simulink model "controlGPI_pos_2dof_conMI"  (R2023b)
settings: Solver=ode45  StartTime=0.0  StopTime=tsim  FixedStep=5e-4  MaxStep=tstep
undefined symbols (not defined in the file): contr_robot_params, ddq, dq, MI_Contr1, MI_Contr2, MI_motor1, MI_motor2, ndof, NN_Bspline_params, NN_RBF_params, nn_select, ns, Pc, q, q0, q_cero, q_eq, robot_params, t_qeq_init, t_tr_init, t_trtr, tau_L, tau_L_mags, tr_muestra, Wc, Zc
libraries: mcbcontrolslib x4, spsRMSLib x4, simulink x2
(part 1 of 2)
settings Model: Creator=HP  LastModifiedBy=HP

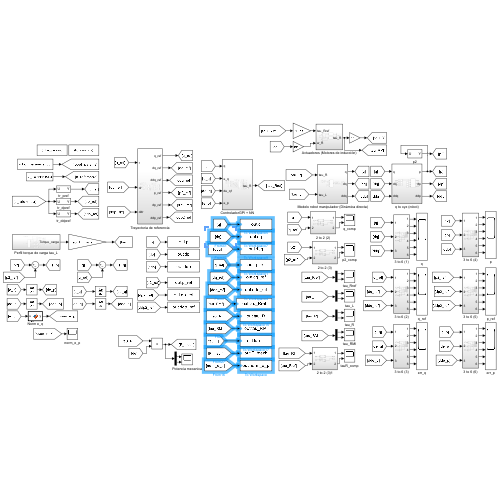
[thumbnail: Simulink's stored preview of the top-level diagram]
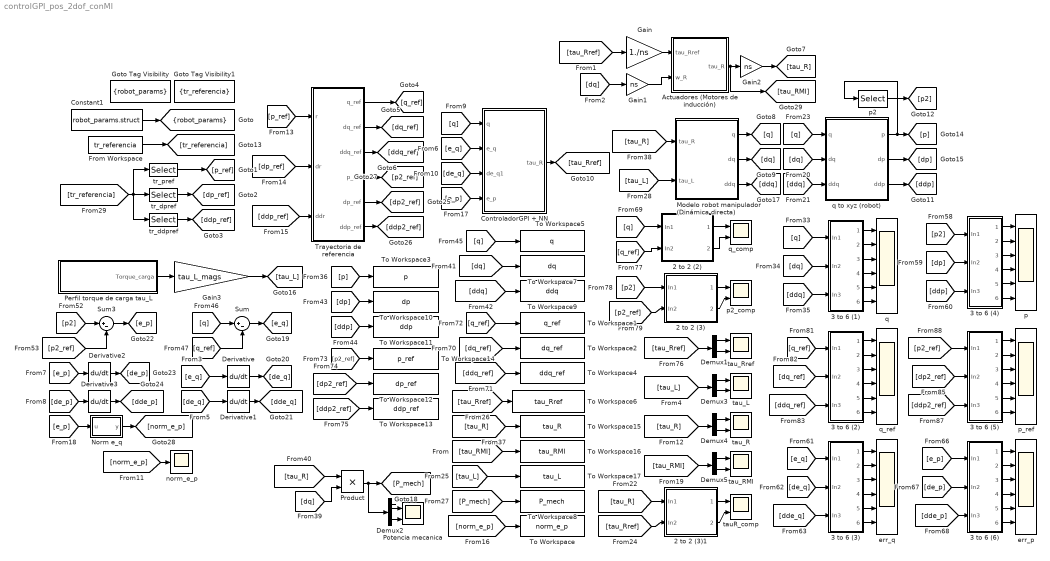
== system controlGPI_pos_2dof_conMI ==
  2 to 2 (2) : Subsystem
  2 to 2 (3) : Subsystem
  2 to 2 (3)1 : Subsystem
  3 to 6 (1) : Subsystem
  3 to 6 (2) : Subsystem
  3 to 6 (3) : Subsystem
  3 to 6 (4) : Subsystem
  3 to 6 (5) : Subsystem
  3 to 6 (6) : Subsystem
  Actuadores (Motores de inducción) : Subsystem
  Constant1 : Constant  Value=robot_params.struct  OutDataTypeStr=Bus: robot_params_bus
  ControladorGPI + NN : Subsystem
  Demux{1..5} (5 alike) : Demux  Outputs=2
  Derivative{,1..3} (4 alike) : Derivative
  From Workspace : FromWorkspace  VariableName=tr_referencia
  Gain : Gain  Gain=1./ns
  Gain1 : Gain  Gain=ns
  Gain2 : Gain  Gain=ns
  Gain3 : Gain  Gain=tau_L_mags
  Goto Tag Visibility : GotoTagVisibility  GotoTag=robot_params
  Goto Tag Visibility1 : GotoTagVisibility  GotoTag=tr_referencia
  Modelo robot manipulador (Dinámica directa) : Subsystem
  Norm e_q : MATLAB Function  TreatAsAtomicUnit=on
  Perfil torque de carga tau_L : Subsystem
  Potencia mecanica : Scope  NumInputPorts=2
  Product : Product
  Sum : Sum  Inputs=|+-
  Sum3 : Sum  Inputs=|+-
  To Workspace : ToWorkspace  VariableName=norm_e_p  SaveFormat=Timeseries  SampleTime=-1
  To Workspace1 : ToWorkspace  VariableName=q_ref  SaveFormat=Timeseries  SampleTime=-1
  To Workspace10 : ToWorkspace  VariableName=dp  SaveFormat=Timeseries  SampleTime=-1
  To Workspace11 : ToWorkspace  VariableName=ddp  SaveFormat=Timeseries  SampleTime=-1
  To Workspace12 : ToWorkspace  VariableName=dp_ref  SaveFormat=Timeseries  SampleTime=-1
  To Workspace13 : ToWorkspace  VariableName=ddp_ref  SaveFormat=Timeseries  SampleTime=-1
  To Workspace14 : ToWorkspace  VariableName=p_ref  SaveFormat=Timeseries  SampleTime=-1
  To Workspace15 : ToWorkspace  VariableName=tau_R  SaveFormat=Timeseries  SampleTime=-1
  To Workspace16 : ToWorkspace  VariableName=tau_RMI  SaveFormat=Timeseries  SampleTime=-1
  To Workspace17 : ToWorkspace  VariableName=tau_L  SaveFormat=Timeseries  SampleTime=-1
  To Workspace2 : ToWorkspace  VariableName=dq_ref  SaveFormat=Timeseries  SampleTime=-1
  To Workspace3 : ToWorkspace  VariableName=p  SaveFormat=Timeseries  SampleTime=-1
  To Workspace4 : ToWorkspace  VariableName=ddq_ref  SaveFormat=Timeseries  SampleTime=-1
  To Workspace5 : ToWorkspace  VariableName=q  SaveFormat=Timeseries  SampleTime=-1
  To Workspace6 : ToWorkspace  VariableName=tau_Rref  SaveFormat=Timeseries  SampleTime=-1
  To Workspace7 : ToWorkspace  VariableName=dq  SaveFormat=Timeseries  SampleTime=-1
  To Workspace8 : ToWorkspace  VariableName=P_mech  SaveFormat=Timeseries  SampleTime=-1
  To Workspace9 : ToWorkspace  VariableName=ddq  SaveFormat=Timeseries  SampleTime=-1
  Trayectoria de referencia : Subsystem
  err_p : Scope  NumInputPorts=6
  err_q : Scope  NumInputPorts=6
  norm_e_p : Scope
  p : Scope  NumInputPorts=6
  p2 : Selector  NumberOfDimensions=2  InputPortWidth=3  IndexOptions=Index vector (dialog),Index vector (dialog)  Indices=[1:2],2  OutputSizes=1,1
  p2_comp : Scope  NumInputPorts=2
  p_ref : Scope  NumInputPorts=6
  q : Scope  NumInputPorts=6
  q to xyz (robot) : Subsystem
  q_comp : Scope  NumInputPorts=2
  q_ref : Scope  NumInputPorts=6
  tauR_comp : Scope  NumInputPorts=2
  tau_L : Scope  NumInputPorts=2
  tau_R : Scope  NumInputPorts=2
  tau_RMI : Scope  NumInputPorts=2
  tau_Rref : Scope  NumInputPorts=2
  tr_ddpref : Selector  NumberOfDimensions=2  InputPortWidth=3  IndexOptions=Index vector (dialog),Index vector (dialog)  Indices=[5:6],1  OutputSizes=1,1
  tr_dpref : Selector  NumberOfDimensions=2  InputPortWidth=3  IndexOptions=Index vector (dialog),Index vector (dialog)  Indices=[3:4],1  OutputSizes=1,1
  tr_pref : Selector  NumberOfDimensions=2  InputPortWidth=3  IndexOptions=Index vector (dialog),Index vector (dialog)  Indices=[1:2],1  OutputSizes=1,1
  tag scope: robot_params=scoped
  wires:
  From Workspace/1 -> [tr_referencia]
  Constant1/1 -> [robot_params]
  [tau_L] -> Modelo robot manipulador (Dinámica directa)/2(tau_L)
  [tau_R] -> Modelo robot manipulador (Dinámica directa)/1(tau_R)
  Modelo robot manipulador (Dinámica directa)/1(q) -> [q]
  Modelo robot manipulador (Dinámica directa)/2(dq) -> [dq]
  Modelo robot manipulador (Dinámica directa)/3(ddq) -> [ddq]
  ControladorGPI + NN/1(tau_R) -> [tau_Rref]
  [tr_referencia] -> tr_ddpref/1, tr_pref/1, tr_dpref/1
  tr_pref/1 -> [p_ref]
  tr_dpref/1 -> [dp_ref]
  tr_ddpref/1 -> [ddp_ref]
  [e_q] -> 3 to 6 (3)/1(In1)
  [dq_ref] -> 3 to 6 (2)/2(In2)
  [dq] -> 3 to 6 (1)/2(In2)
  2 to 2 (3)/1(1) -> p2_comp/1
  [tau_R] -> Product/1
  Product/1 -> Demux2/1, [P_mech]
  [q] -> 3 to 6 (1)/1(In1)
  [p2] -> 2 to 2 (3)/1(In1)
  [ddq_ref] -> 3 to 6 (2)/3(In3)
  3 to 6 (1)/5(Out5) -> q/5
  Demux2/1 -> Potencia mecanica/1
  [dde_p] -> 3 to 6 (6)/3(In3)
  [p2] -> 3 to 6 (4)/1(In1)
  Demux2/2 -> Potencia mecanica/2
  Demux1/2 -> tau_Rref/2
  3 to 6 (1)/6(Out6) -> q/6
  [de_q] -> 3 to 6 (3)/2(In2)
  [e_p] -> 3 to 6 (6)/1(In1)
  [dq] -> Product/2
  3 to 6 (1)/1(Out1) -> q/1
  [de_p] -> 3 to 6 (6)/2(In2)
  3 to 6 (1)/2(Out2) -> q/2
  [q_ref] -> 2 to 2 (2)/2(In2)
  [tau_Rref] -> Demux1/1
  [ddq] -> 3 to 6 (1)/3(In3)
  [p2_ref] -> 2 to 2 (3)/2(In2)
  [dde_q] -> 3 to 6 (3)/3(In3)
  3 to 6 (1)/4(Out4) -> q/4
  [q_ref] -> 3 to 6 (2)/1(In1)
  [ddp] -> 3 to 6 (4)/3(In3)
  [dp] -> 3 to 6 (4)/2(In2)
  Demux1/1 -> tau_Rref/1
  3 to 6 (1)/3(Out3) -> q/3
  q to xyz (robot)/1(p) -> [p], p2/1
  [dq] -> q to xyz (robot)/2(dq)
  Derivative/1 -> [de_q]
  [ddq] -> q to xyz (robot)/3(ddq)
  [q] -> To Workspace5/1
  [tau_Rref] -> To Workspace6/1
  [dq_ref] -> To Workspace2/1
  [p2_ref] -> Sum3/2
  [q] -> q to xyz (robot)/1(q)
  [ddq] -> To Workspace9/1
  [p2_ref] -> To Workspace14/1
  [q] -> Sum/1
  [ddq_ref] -> To Workspace4/1
  Sum3/1 -> [e_p]
  [q_ref] -> To Workspace1/1
  [q_ref] -> Sum/2
  [p2] -> Sum3/1
  q to xyz (robot)/2(dp) -> [dp]
  [dp] -> To Workspace10/1
  Derivative1/1 -> [dde_q]
  [dp2_ref] -> To Workspace12/1
  q to xyz (robot)/3(ddp) -> [ddp]
  [P_mech] -> To Workspace8/1
  [ddp] -> To Workspace11/1
  [p] -> To Workspace3/1
  [dq] -> To Workspace7/1
  Sum/1 -> [e_q]
  p2/1 -> [p2]
  [ddp2_ref] -> To Workspace13/1
  2 to 2 (2)/1(1) -> q_comp/1
  2 to 2 (2)/2(2) -> q_comp/2
  3 to 6 (2)/4(Out4) -> q_ref/4
  3 to 6 (2)/6(Out6) -> q_ref/6
  3 to 6 (2)/3(Out3) -> q_ref/3
  3 to 6 (2)/1(Out1) -> q_ref/1
  3 to 6 (2)/2(Out2) -> q_ref/2
  3 to 6 (2)/5(Out5) -> q_ref/5
  3 to 6 (3)/4(Out4) -> err_q/4
  3 to 6 (3)/6(Out6) -> err_q/6
  3 to 6 (3)/3(Out3) -> err_q/3
  3 to 6 (3)/1(Out1) -> err_q/1
  3 to 6 (3)/2(Out2) -> err_q/2
  3 to 6 (3)/5(Out5) -> err_q/5
  3 to 6 (4)/4(Out4) -> p/4
  3 to 6 (4)/6(Out6) -> p/6
  3 to 6 (4)/3(Out3) -> p/3
  3 to 6 (4)/1(Out1) -> p/1
  3 to 6 (4)/2(Out2) -> p/2
  3 to 6 (4)/5(Out5) -> p/5
  3 to 6 (5)/4(Out4) -> p_ref/4
  3 to 6 (5)/6(Out6) -> p_ref/6
  3 to 6 (5)/3(Out3) -> p_ref/3
  3 to 6 (5)/1(Out1) -> p_ref/1
  3 to 6 (5)/2(Out2) -> p_ref/2
  3 to 6 (5)/5(Out5) -> p_ref/5
  [p2_ref] -> 3 to 6 (5)/1(In1)
  [dp2_ref] -> 3 to 6 (5)/2(In2)
  [ddp2_ref] -> 3 to 6 (5)/3(In3)
  3 to 6 (6)/4(Out4) -> err_p/4
  3 to 6 (6)/6(Out6) -> err_p/6
  3 to 6 (6)/3(Out3) -> err_p/3
  3 to 6 (6)/1(Out1) -> err_p/1
  3 to 6 (6)/2(Out2) -> err_p/2
  3 to 6 (6)/5(Out5) -> err_p/5
  2 to 2 (3)/2(2) -> p2_comp/2
  Norm e_q/1(y) -> [norm_e_p]
  [norm_e_p] -> To Workspace/1
  [e_p] -> Norm e_q/1(u)
  [e_p] -> ControladorGPI + NN/4(e_p)
  [q] -> 2 to 2 (2)/1(In1)
  [e_q] -> ControladorGPI + NN/2(e_q)
  Demux3/2 -> tau_L/2
  Demux3/1 -> tau_L/1
  [tau_L] -> Demux3/1
  [e_q] -> Derivative/1
  [de_q] -> Derivative1/1
  Derivative2/1 -> [de_p]
  [e_p] -> Derivative2/1
  Derivative3/1 -> [dde_p]
  [de_p] -> Derivative3/1
  [q] -> ControladorGPI + NN/1(q)
  [de_q] -> ControladorGPI + NN/3(de_q1)
  [norm_e_p] -> norm_e_p/1
  Trayectoria de referencia/6(ddp_ref) -> [ddp2_ref]
  Trayectoria de referencia/5(dp_ref) -> [dp2_ref]
  Trayectoria de referencia/1(q_ref) -> [q_ref]
  [dp_ref] -> Trayectoria de referencia/2(dr)
  Trayectoria de referencia/3(ddq_ref) -> [ddq_ref]
  Trayectoria de referencia/2(dq_ref) -> [dq_ref]
  [p_ref] -> Trayectoria de referencia/1(r)
  [ddp_ref] -> Trayectoria de referencia/3(ddr)
  Trayectoria de referencia/4(p_ref) -> [p2_ref]
  Actuadores (Motores de inducción)/1(tau_R) -> [tau_RMI], Gain2/1
  Gain2/1 -> [tau_R]
  Gain1/1 -> Actuadores (Motores de inducción)/2(w_R)
  Gain/1 -> Actuadores (Motores de inducción)/1(tau_Rref)
  [tau_Rref] -> Gain/1
  [dq] -> Gain1/1
  [tau_R] -> To Workspace15/1
  Demux4/1 -> tau_R/1
  [tau_R] -> Demux4/1
  Demux4/2 -> tau_R/2
  Demux5/1 -> tau_RMI/1
  [tau_RMI] -> Demux5/1
  Demux5/2 -> tau_RMI/2
  2 to 2 (3)1/1(1) -> tauR_comp/1
  2 to 2 (3)1/2(2) -> tauR_comp/2
  [tau_R] -> 2 to 2 (3)1/1(In1)
  [tau_Rref] -> 2 to 2 (3)1/2(In2)
  [tau_RMI] -> To Workspace16/1
  Perfil torque de carga tau_L/1(Torque_carga) -> Gain3/1
  Gain3/1 -> [tau_L]
  [tau_L] -> To Workspace17/1

== system controlGPI_pos_2dof_conMI/2 to 2 (2) ==
  In1 : Inport
  In2 : Inport  Port=2
  Demux3 : Demux  Outputs=2
  Demux4 : Demux  Outputs=2
  Mux8 : Mux  Inputs=2
  Mux9 : Mux  Inputs=2
  1 : Outport
  2 : Outport  Port=2
  wires:
  Demux3/1 -> Mux8/1
  Demux3/2 -> Mux9/1
  Mux9/1 -> 2/1
  Demux4/2 -> Mux9/2
  Demux4/1 -> Mux8/2
  Mux8/1 -> 1/1
  In1/1 -> Demux3/1
  In2/1 -> Demux4/1

== system controlGPI_pos_2dof_conMI/2 to 2 (3) ==
  In1 : Inport
  In2 : Inport  Port=2
  Demux3 : Demux  Outputs=2
  Demux4 : Demux  Outputs=2
  Mux8 : Mux  Inputs=2
  Mux9 : Mux  Inputs=2
  1 : Outport
  2 : Outport  Port=2
  wires:
  Demux3/1 -> Mux8/1
  Demux3/2 -> Mux9/1
  Mux9/1 -> 2/1
  Demux4/2 -> Mux9/2
  Demux4/1 -> Mux8/2
  Mux8/1 -> 1/1
  In1/1 -> Demux3/1
  In2/1 -> Demux4/1

== system controlGPI_pos_2dof_conMI/2 to 2 (3)1 ==
  In1 : Inport
  In2 : Inport  Port=2
  Demux3 : Demux  Outputs=2
  Demux4 : Demux  Outputs=2
  Mux8 : Mux  Inputs=2
  Mux9 : Mux  Inputs=2
  1 : Outport
  2 : Outport  Port=2
  wires:
  Demux3/1 -> Mux8/1
  Demux3/2 -> Mux9/1
  Mux9/1 -> 2/1
  Demux4/2 -> Mux9/2
  Demux4/1 -> Mux8/2
  Mux8/1 -> 1/1
  In1/1 -> Demux3/1
  In2/1 -> Demux4/1

== system controlGPI_pos_2dof_conMI/3 to 6 (1) ==
  In1 : Inport
  In2 : Inport  Port=2
  In3 : Inport  Port=3
  Demux2 : Demux  Outputs=2
  Demux3 : Demux  Outputs=2
  Demux4 : Demux  Outputs=2
  Out1 : Outport
  Out2 : Outport  Port=2
  Out3 : Outport  Port=3
  Out4 : Outport  Port=4
  Out5 : Outport  Port=5
  Out6 : Outport  Port=6
  wires:
  In3/1 -> Demux4/1
  Demux4/1 -> Out3/1
  Demux2/1 -> Out1/1
  Demux3/2 -> Out5/1
  Demux3/1 -> Out2/1
  In1/1 -> Demux2/1
  Demux4/2 -> Out6/1
  Demux2/2 -> Out4/1
  In2/1 -> Demux3/1

== system controlGPI_pos_2dof_conMI/3 to 6 (2) ==
  In1 : Inport
  In2 : Inport  Port=2
  In3 : Inport  Port=3
  Demux2 : Demux  Outputs=2
  Demux3 : Demux  Outputs=2
  Demux4 : Demux  Outputs=2
  Out1 : Outport
  Out2 : Outport  Port=2
  Out3 : Outport  Port=3
  Out4 : Outport  Port=4
  Out5 : Outport  Port=5
  Out6 : Outport  Port=6
  wires:
  In3/1 -> Demux4/1
  Demux4/1 -> Out3/1
  Demux2/1 -> Out1/1
  Demux3/2 -> Out5/1
  Demux3/1 -> Out2/1
  In1/1 -> Demux2/1
  Demux4/2 -> Out6/1
  Demux2/2 -> Out4/1
  In2/1 -> Demux3/1

== system controlGPI_pos_2dof_conMI/3 to 6 (3) ==
  In1 : Inport
  In2 : Inport  Port=2
  In3 : Inport  Port=3
  Demux2 : Demux  Outputs=2
  Demux3 : Demux  Outputs=2
  Demux4 : Demux  Outputs=2
  Out1 : Outport
  Out2 : Outport  Port=2
  Out3 : Outport  Port=3
  Out4 : Outport  Port=4
  Out5 : Outport  Port=5
  Out6 : Outport  Port=6
  wires:
  In3/1 -> Demux4/1
  Demux4/1 -> Out3/1
  Demux2/1 -> Out1/1
  Demux3/2 -> Out5/1
  Demux3/1 -> Out2/1
  In1/1 -> Demux2/1
  Demux4/2 -> Out6/1
  Demux2/2 -> Out4/1
  In2/1 -> Demux3/1

== system controlGPI_pos_2dof_conMI/3 to 6 (4) ==
  In1 : Inport
  In2 : Inport  Port=2
  In3 : Inport  Port=3
  Demux2 : Demux  Outputs=2
  Demux3 : Demux  Outputs=2
  Demux4 : Demux  Outputs=2
  Out1 : Outport
  Out2 : Outport  Port=2
  Out3 : Outport  Port=3
  Out4 : Outport  Port=4
  Out5 : Outport  Port=5
  Out6 : Outport  Port=6
  wires:
  In3/1 -> Demux4/1
  Demux4/1 -> Out3/1
  Demux2/1 -> Out1/1
  Demux3/2 -> Out5/1
  Demux3/1 -> Out2/1
  In1/1 -> Demux2/1
  Demux4/2 -> Out6/1
  Demux2/2 -> Out4/1
  In2/1 -> Demux3/1

== system controlGPI_pos_2dof_conMI/3 to 6 (5) ==
  In1 : Inport
  In2 : Inport  Port=2
  In3 : Inport  Port=3
  Demux2 : Demux  Outputs=2
  Demux3 : Demux  Outputs=2
  Demux4 : Demux  Outputs=2
  Out1 : Outport
  Out2 : Outport  Port=2
  Out3 : Outport  Port=3
  Out4 : Outport  Port=4
  Out5 : Outport  Port=5
  Out6 : Outport  Port=6
  wires:
  In3/1 -> Demux4/1
  Demux4/1 -> Out3/1
  Demux2/1 -> Out1/1
  Demux3/2 -> Out5/1
  Demux3/1 -> Out2/1
  In1/1 -> Demux2/1
  Demux4/2 -> Out6/1
  Demux2/2 -> Out4/1
  In2/1 -> Demux3/1

== system controlGPI_pos_2dof_conMI/3 to 6 (6) ==
  In1 : Inport
  In2 : Inport  Port=2
  In3 : Inport  Port=3
  Demux2 : Demux  Outputs=2
  Demux3 : Demux  Outputs=2
  Demux4 : Demux  Outputs=2
  Out1 : Outport
  Out2 : Outport  Port=2
  Out3 : Outport  Port=3
  Out4 : Outport  Port=4
  Out5 : Outport  Port=5
  Out6 : Outport  Port=6
  wires:
  In3/1 -> Demux4/1
  Demux4/1 -> Out3/1
  Demux2/1 -> Out1/1
  Demux3/2 -> Out5/1
  Demux3/1 -> Out2/1
  In1/1 -> Demux2/1
  Demux4/2 -> Out6/1
  Demux2/2 -> Out4/1
  In2/1 -> Demux3/1

== system controlGPI_pos_2dof_conMI/Actuadores (Motores de inducción) ==
  tau_Rref : Inport
  w_R : Inport  Port=2
  Demux : Demux  Outputs=2
  Demux3 : Demux  Outputs=2
  MI1 + PBC Torque Controller : Subsystem
  MI2 + PBC Torque Controller : Subsystem
  Mux : Mux  Inputs=2
  tau_R : Outport
  wires:
  Demux3/1 -> MI1 + PBC Torque Controller/2(dq)
  Demux/1 -> MI1 + PBC Torque Controller/1(tau_Rref)
  MI1 + PBC Torque Controller/1(tau_R) -> Mux/1
  MI2 + PBC Torque Controller/1(tau_R) -> Mux/2
  Demux3/2 -> MI2 + PBC Torque Controller/2(dq)
  Demux/2 -> MI2 + PBC Torque Controller/1(tau_Rref)
  tau_Rref/1 -> Demux/1
  w_R/1 -> Demux3/1
  Mux/1 -> tau_R/1

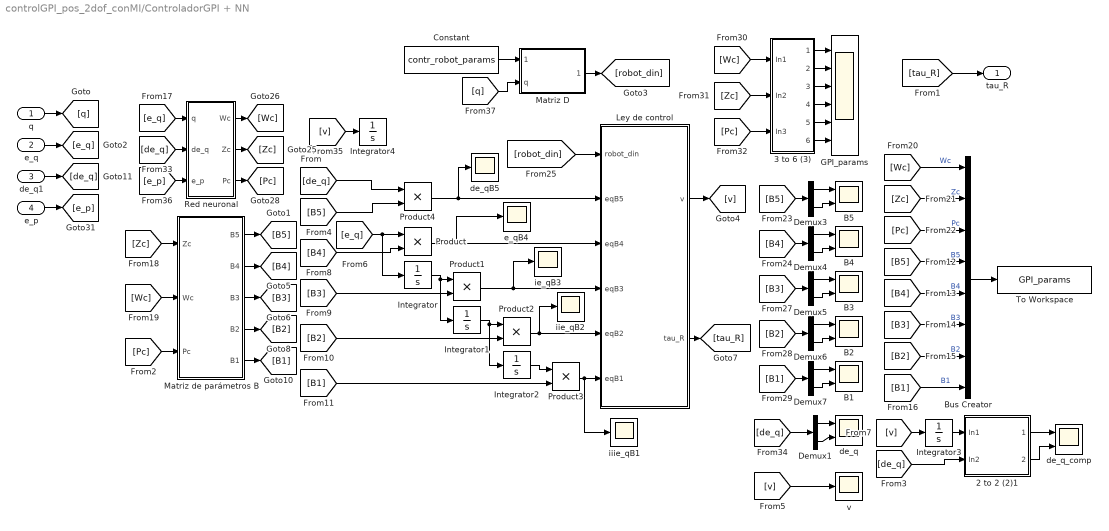
== system controlGPI_pos_2dof_conMI/ControladorGPI + NN ==
  q : Inport
  e_q : Inport  Port=2
  de_q1 : Inport  Port=3
  e_p : Inport  Port=4
  2 to 2 (2)1 : Subsystem
  3 to 6 (3) : Subsystem
  B{1..5} (5 alike) : Scope  NumInputPorts=2
  Bus Creator : BusCreator  Inputs=8
  Constant : Constant  Value=contr_robot_params  OutDataTypeStr=Bus: robot_params_bus
  Demux{1,3..7} (6 alike) : Demux  Outputs=2
  GPI_params : Scope  NumInputPorts=6
  Integrator{,1..4} (5 alike) : Integrator
  Ley de control : MATLAB Function  TreatAsAtomicUnit=on
  Matriz D : MATLAB Function  TreatAsAtomicUnit=on
  Matriz de parámetros B : MATLAB Function  TreatAsAtomicUnit=on
  Product{,1..4} (5 alike) : Product
  Red neuronal : Subsystem
  To Workspace : ToWorkspace  VariableName=GPI_params  SaveFormat=Timeseries  SampleTime=-1
  de_q : Scope  NumInputPorts=2
  de_qB5 : Scope
  de_q_comp : Scope  NumInputPorts=2
  e_qB4 : Scope
  ie_qB3 : Scope
  iie_qB2 : Scope
  iiie_qB1 : Scope
  v : Scope
  tau_R : Outport
  wires:
  Ley de control/2(tau_R) -> [tau_R]
  [tau_R] -> tau_R/1
  e_q/1 -> [e_q]
  [e_q] -> Integrator/1, Product/1
  Integrator/1 -> Integrator1/1, Product1/1
  Integrator1/1 -> Integrator2/1, Product2/1
  Integrator2/1 -> Product3/1
  Product3/1 -> iiie_qB1/1, Ley de control/6(eqB1)
  Product2/1 -> iie_qB2/1, Ley de control/5(eqB2)
  Product1/1 -> ie_qB3/1, Ley de control/4(eqB3)
  Product/1 -> e_qB4/1, Ley de control/3(eqB4)
  Ley de control/1(v) -> [v]
  Product4/1 -> de_qB5/1, Ley de control/2(eqB5)
  [Zc] -> Matriz de parámetros B/1(Zc)
  [Wc] -> Matriz de parámetros B/2(Wc)
  [Pc] -> Matriz de parámetros B/3(Pc)
  Matriz de parámetros B/1(B5) -> [B5]
  Matriz de parámetros B/2(B4) -> [B4]
  Matriz de parámetros B/3(B3) -> [B3]
  Matriz de parámetros B/4(B2) -> [B2]
  Matriz de parámetros B/5(B1) -> [B1]
  [B5] -> Product4/2
  [B4] -> Product/2
  [B3] -> Product1/2
  [B2] -> Product2/2
  [B1] -> Product3/2
  Bus Creator/1 -> To Workspace/1
  [Wc] -> Bus Creator/1  "Wc"
  [Zc] -> Bus Creator/2  "Zc"
  [Pc] -> Bus Creator/3  "Pc"
  [B5] -> Bus Creator/4  "B5"
  [B4] -> Bus Creator/5  "B4"
  [B3] -> Bus Creator/6  "B3"
  [B2] -> Bus Creator/7  "B2"
  [B1] -> Bus Creator/8  "B1"
  Demux3/2 -> B5/2
  Demux3/1 -> B5/1
  [B5] -> Demux3/1
  Demux4/2 -> B4/2
  Demux4/1 -> B4/1
  [B4] -> Demux4/1
  Demux5/1 -> B3/1
  Demux5/2 -> B3/2
  [B3] -> Demux5/1
  Demux6/1 -> B2/1
  Demux6/2 -> B2/2
  [B2] -> Demux6/1
  Demux7/1 -> B1/1
  Demux7/2 -> B1/2
  [B1] -> Demux7/1
  Red neuronal/2(Zc) -> [Zc]
  Red neuronal/1(Wc) -> [Wc]
  Red neuronal/3(Pc) -> [Pc]
  [de_q] -> Red neuronal/2(de_q)
  [Wc] -> 3 to 6 (3)/1(In1)
  [Zc] -> 3 to 6 (3)/2(In2)
  [Pc] -> 3 to 6 (3)/3(In3)
  3 to 6 (3)/4(Out4) -> GPI_params/4
  3 to 6 (3)/2(Out2) -> GPI_params/2
  3 to 6 (3)/3(Out3) -> GPI_params/3
  3 to 6 (3)/5(Out5) -> GPI_params/5
  3 to 6 (3)/1(Out1) -> GPI_params/1
  3 to 6 (3)/6(Out6) -> GPI_params/6
  [e_q] -> Red neuronal/1(q)
  [de_q] -> Demux1/1
  Demux1/1 -> de_q/1
  Demux1/2 -> de_q/2
  de_q1/1 -> [de_q]
  e_p/1 -> [e_p]
  [e_p] -> Red neuronal/3(e_p)
  [robot_din] -> Ley de control/1(robot_din)
  q/1 -> [q]
  [v] -> Integrator3/1
  Integrator3/1 -> 2 to 2 (2)1/1(In1)
  [de_q] -> 2 to 2 (2)1/2(In2)
  2 to 2 (2)1/1(1) -> de_q_comp/1
  2 to 2 (2)1/2(2) -> de_q_comp/2
  [v] -> v/1
  [v] -> Integrator4/1
  [de_q] -> Product4/1
  Matriz D/1(robot_din) -> [robot_din]
  [q] -> Matriz D/2(q)
  Constant/1 -> Matriz D/1(robot_params)

== system controlGPI_pos_2dof_conMI/Modelo robot manipulador (Dinámica directa) ==
  tau_R : Inport
  tau_L : Inport  Port=2
  Dinámica directa : MATLAB Function  TreatAsAtomicUnit=on
  int_ddq : Integrator  InitialCondition=q_cero
  int_dq : Integrator  InitialCondition=q_eq
  q : Outport
  dq : Outport  Port=2
  ddq : Outport  Port=3
  wires:
  [tau_L] -> Dinámica directa/5(tau_L)
  int_ddq/1 -> [dq], int_dq/1
  [robot_params] -> Dinámica directa/1(robot_params)
  [dq] -> Dinámica directa/3(dq)
  int_dq/1 -> [q]
  [tau_R] -> Dinámica directa/4(tau_R)
  Dinámica directa/1(ddq) -> int_ddq/1, [ddq]
  [q] -> q/1
  [dq] -> dq/1
  [ddq] -> ddq/1
  tau_R/1 -> [tau_R]
  tau_L/1 -> [tau_L]
  [q] -> Dinámica directa/2(q)

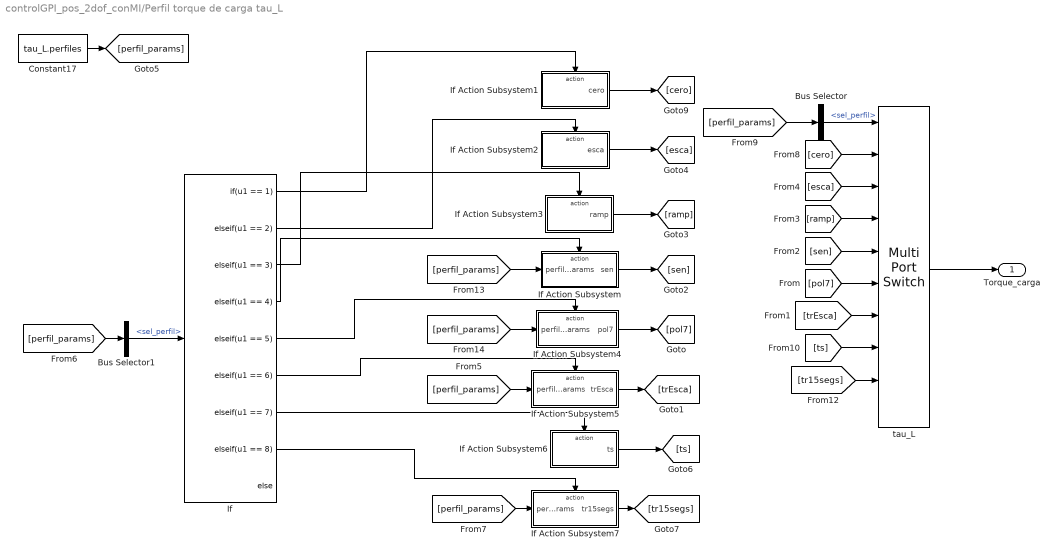
== system controlGPI_pos_2dof_conMI/Perfil torque de carga tau_L ==
  Bus Selector : BusSelector  OutputSignals=sel_perfil
  Bus Selector1 : BusSelector  OutputSignals=sel_perfil
  Constant17 : Constant  Value=tau_L.perfiles  OutDataTypeStr=Bus: Perfil_bus
  If : If  IfExpression=u1 == 1  ElseIfExpressions=u1 == 2,u1 == 3,u1 == 4,u1 == 5,u1 == 6,u1 == 7,u1 == 8
  If Action Subsystem : Subsystem  TreatAsAtomicUnit=on
  If Action Subsystem1 : Subsystem  TreatAsAtomicUnit=on
  If Action Subsystem2 : Subsystem  TreatAsAtomicUnit=on
  If Action Subsystem3 : Subsystem  TreatAsAtomicUnit=on
  If Action Subsystem4 : Subsystem  TreatAsAtomicUnit=on
  If Action Subsystem5 : Subsystem  TreatAsAtomicUnit=on
  If Action Subsystem6 : Subsystem  TreatAsAtomicUnit=on
  If Action Subsystem7 : Subsystem  TreatAsAtomicUnit=on
  tau_L : MultiPortSwitch  Inputs=9  SaturateOnIntegerOverflow=off  InputSameDT=off
  Torque_carga : Outport
  wires:
  tau_L/1 -> Torque_carga/1
  [ramp] -> tau_L/4
  [trEsca] -> tau_L/7
  [pol7] -> tau_L/6
  [sen] -> tau_L/5
  [esca] -> tau_L/3
  Constant17/1 -> [perfil_params]
  [ts] -> tau_L/8
  [tr15segs] -> tau_L/9
  Bus Selector/1 -> tau_L/1  "<sel_perfil>"
  [perfil_params] -> Bus Selector/1
  If Action Subsystem/1(sen) -> [sen]
  [perfil_params] -> Bus Selector1/1
  Bus Selector1/1 -> If/1  "<sel_perfil>"
  If/4 -> If Action Subsystem/Action
  If Action Subsystem1/1(cero) -> [cero]
  [cero] -> tau_L/2
  [perfil_params] -> If Action Subsystem/1(perfil_params)
  If/1 -> If Action Subsystem1/Action
  If Action Subsystem2/1(esca) -> [esca]
  If/2 -> If Action Subsystem2/Action
  If Action Subsystem3/1(ramp) -> [ramp]
  If/3 -> If Action Subsystem3/Action
  [perfil_params] -> If Action Subsystem4/1(perfil_params)
  If/5 -> If Action Subsystem4/Action
  If Action Subsystem4/1(pol7) -> [pol7]
  If Action Subsystem5/1(trEsca) -> [trEsca]
  [perfil_params] -> If Action Subsystem5/1(perfil_params)
  If Action Subsystem6/1(ts) -> [ts]
  If/6 -> If Action Subsystem5/Action
  If/7 -> If Action Subsystem6/Action
  If Action Subsystem7/1(tr15segs) -> [tr15segs]
  If/8 -> If Action Subsystem7/Action
  [perfil_params] -> If Action Subsystem7/1(perfil_params)

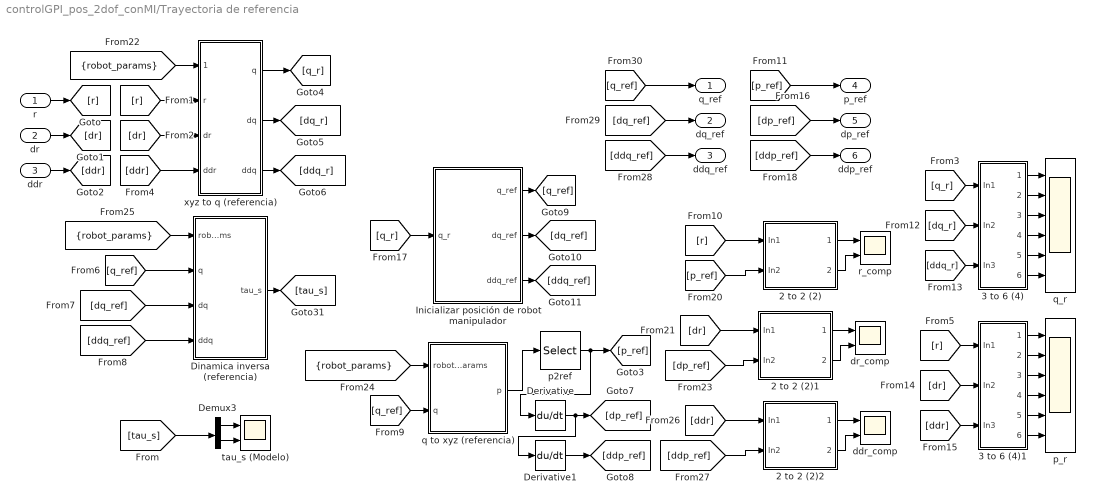
== system controlGPI_pos_2dof_conMI/Trayectoria de referencia ==
  r : Inport
  dr : Inport  Port=2
  ddr : Inport  Port=3
  2 to 2 (2) : Subsystem
  2 to 2 (2)1 : Subsystem
  2 to 2 (2)2 : Subsystem
  3 to 6 (4) : Subsystem
  3 to 6 (4)1 : Subsystem
  Demux3 : Demux  Outputs=2
  Derivative : Derivative
  Derivative1 : Derivative
  Dinamica inversa (referencia) : MATLAB Function  TreatAsAtomicUnit=on
  Inicializar posición de robot manipulador : Subsystem
  ddr_comp : Scope  NumInputPorts=2
  dr_comp : Scope  NumInputPorts=2
  p2ref : Selector  NumberOfDimensions=2  InputPortWidth=3  IndexOptions=Index vector (dialog),Index vector (dialog)  Indices=[1:2],2  OutputSizes=1,1
  p_r : Scope  NumInputPorts=6
  q to xyz (referencia) : MATLAB Function  TreatAsAtomicUnit=on
  q_r : Scope  NumInputPorts=6
  r_comp : Scope  NumInputPorts=2
  tau_s (Modelo) : Scope  NumInputPorts=2
  xyz to q (referencia) : MATLAB Function  TreatAsAtomicUnit=on
  q_ref : Outport
  dq_ref : Outport  Port=2
  ddq_ref : Outport  Port=3
  p_ref : Outport  Port=4
  dp_ref : Outport  Port=5
  ddp_ref : Outport  Port=6
  wires:
  xyz to q (referencia)/1(q) -> [q_r]
  [robot_params] -> xyz to q (referencia)/1(robot_params)
  [dq_ref] -> Dinamica inversa (referencia)/3(dq)
  [q_ref] -> Dinamica inversa (referencia)/2(q)
  [q_ref] -> q to xyz (referencia)/2(q)
  [r] -> xyz to q (referencia)/2(r)
  xyz to q (referencia)/2(dq) -> [dq_r]
  q to xyz (referencia)/1(p) -> p2ref/1
  [robot_params] -> Dinamica inversa (referencia)/1(robot_params)
  Dinamica inversa (referencia)/1(tau_s) -> [tau_s]
  xyz to q (referencia)/3(ddq) -> [ddq_r]
  [ddq_ref] -> Dinamica inversa (referencia)/4(ddq)
  [ddr] -> xyz to q (referencia)/4(ddr)
  [dr] -> xyz to q (referencia)/3(dr)
  r/1 -> [r]
  dr/1 -> [dr]
  ddr/1 -> [ddr]
  Derivative/1 -> Derivative1/1, [dp_ref]
  [tau_s] -> Demux3/1
  [q_r] -> Inicializar posición de robot manipulador/1(q_r)
  [robot_params] -> q to xyz (referencia)/1(robot_params)
  p2ref/1 -> [p_ref], Derivative/1
  [r] -> 2 to 2 (2)/1(In1)
  [p_ref] -> p_ref/1
  Derivative1/1 -> [ddp_ref]
  [dp_ref] -> dp_ref/1
  [ddp_ref] -> ddp_ref/1
  [p_ref] -> 2 to 2 (2)/2(In2)
  [dp_ref] -> 2 to 2 (2)1/2(In2)
  [dr] -> 2 to 2 (2)1/1(In1)
  [ddp_ref] -> 2 to 2 (2)2/2(In2)
  [ddr] -> 2 to 2 (2)2/1(In1)
  Inicializar posición de robot manipulador/1(q_ref) -> [q_ref]
  Inicializar posición de robot manipulador/2(dq_ref) -> [dq_ref]
  Inicializar posición de robot manipulador/3(ddq_ref) -> [ddq_ref]
  [ddq_ref] -> ddq_ref/1
  [dq_ref] -> dq_ref/1
  [q_ref] -> q_ref/1
  [ddr] -> 3 to 6 (4)1/3(In3)
  [dq_r] -> 3 to 6 (4)/2(In2)
  [r] -> 3 to 6 (4)1/1(In1)
  [q_r] -> 3 to 6 (4)/1(In1)
  [dr] -> 3 to 6 (4)1/2(In2)
  [ddq_r] -> 3 to 6 (4)/3(In3)
  2 to 2 (2)/1(1) -> r_comp/1
  2 to 2 (2)/2(2) -> r_comp/2
  2 to 2 (2)1/1(1) -> dr_comp/1
  2 to 2 (2)1/2(2) -> dr_comp/2
  2 to 2 (2)2/1(1) -> ddr_comp/1
  2 to 2 (2)2/2(2) -> ddr_comp/2
  3 to 6 (4)/1(Out1) -> q_r/1
  3 to 6 (4)/6(Out6) -> q_r/6
  3 to 6 (4)/5(Out5) -> q_r/5
  3 to 6 (4)/2(Out2) -> q_r/2
  3 to 6 (4)/3(Out3) -> q_r/3
  3 to 6 (4)/4(Out4) -> q_r/4
  3 to 6 (4)1/1(Out1) -> p_r/1
  3 to 6 (4)1/6(Out6) -> p_r/6
  3 to 6 (4)1/5(Out5) -> p_r/5
  3 to 6 (4)1/2(Out2) -> p_r/2
  3 to 6 (4)1/3(Out3) -> p_r/3
  3 to 6 (4)1/4(Out4) -> p_r/4
  Demux3/1 -> tau_s (Modelo)/1
  Demux3/2 -> tau_s (Modelo)/2

== system controlGPI_pos_2dof_conMI/q to xyz (robot) ==
  q : Inport
  dq : Inport  Port=2
  ddq : Inport  Port=3
  Data Store Memory : DataStoreMemory  DataStoreName=q  WriteAfterWriteMsg=warning  InitialValue=zeros(size(q(:,1)))  ShowAdditionalParam=off
  Data Store Memory1 : DataStoreMemory  DataStoreName=dq  WriteAfterWriteMsg=warning  InitialValue=zeros(size(dq(:,1)))  ShowAdditionalParam=off
  Data Store Memory2 : DataStoreMemory  DataStoreName=ddq  WriteAfterWriteMsg=warning  InitialValue=zeros(size(ddq(:,1)))  ShowAdditionalParam=off
  Data Store Read : DataStoreRead  DataStoreName=q  IndexOptions=Index vector (dialog)  Indices=1  OutputSizes=1
  Data Store Read1 : DataStoreRead  DataStoreName=dq  IndexOptions=Index vector (dialog)  Indices=1  OutputSizes=1
  Data Store Read2 : DataStoreRead  DataStoreName=ddq  IndexOptions=Index vector (dialog)  Indices=1  OutputSizes=1
  Data Store Write : DataStoreWrite  DataStoreName=q  IndexOptions=Index vector (dialog)  Indices=1  OutputSizes=1
  Data Store Write1 : DataStoreWrite  DataStoreName=dq  IndexOptions=Index vector (dialog)  Indices=1  OutputSizes=1
  Data Store Write2 : DataStoreWrite  DataStoreName=ddq  IndexOptions=Index vector (dialog)  Indices=1  OutputSizes=1
  q to xyz (referencia) : MATLAB Function  TreatAsAtomicUnit=on
  p : Outport
  dp : Outport  Port=2
  ddp : Outport  Port=3
  wires:
  q/1 -> Data Store Write/1
  ddq/1 -> Data Store Write2/1
  dq/1 -> Data Store Write1/1
  Data Store Read/1 -> q to xyz (referencia)/2(q)
  Data Store Read1/1 -> q to xyz (referencia)/3(dq)
  Data Store Read2/1 -> q to xyz (referencia)/4(ddq)
  q to xyz (referencia)/1(p) -> p/1
  q to xyz (referencia)/2(dp) -> dp/1
  q to xyz (referencia)/3(ddp) -> ddp/1
  [robot_params] -> q to xyz (referencia)/1(robot_params)

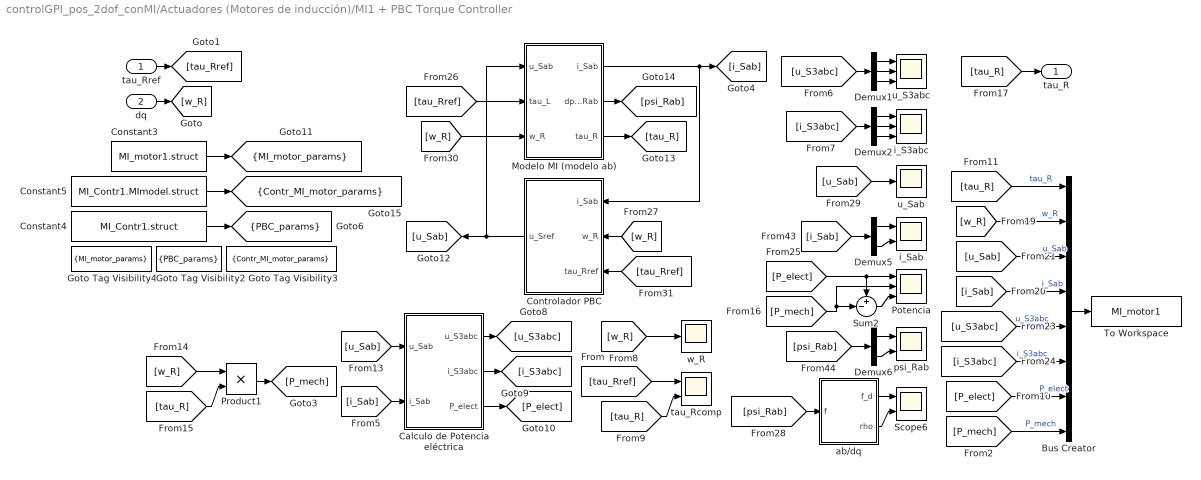
== system controlGPI_pos_2dof_conMI/Actuadores (Motores de inducción)/MI1 + PBC Torque Controller ==
  tau_Rref : Inport
  dq : Inport  Port=2
  Bus Creator : BusCreator  Inputs=8
  Calculo de Potencia eléctrica : Subsystem
  Constant3 : Constant  Value=MI_motor1.struct  OutDataTypeStr=Bus: MI_bus
  Constant4 : Constant  Value=MI_Contr1.struct  OutDataTypeStr=Bus: Contr_bus
  Constant5 : Constant  Value=MI_Contr1.MImodel.struct  OutDataTypeStr=Bus: MI_bus
  Controlador PBC : Subsystem
  Demux1 : Demux  Outputs=3
  Demux2 : Demux  Outputs=3
  Demux5 : Demux  Outputs=2
  Demux6 : Demux  Outputs=2
  Goto Tag Visibility2 : GotoTagVisibility  GotoTag=PBC_params
  Goto Tag Visibility3 : GotoTagVisibility  GotoTag=Contr_MI_motor_params
  Goto Tag Visibility4 : GotoTagVisibility  GotoTag=MI_motor_params
  Modelo MI (modelo ab) : Subsystem
  Potencia : Scope  NumInputPorts=3
  Product1 : Product
  Scope6 : Scope  NumInputPorts=2
  Sum2 : Sum  Inputs=+-|
  To Workspace : ToWorkspace  VariableName=MI_motor1  SaveFormat=Timeseries  SampleTime=-1
  ab/dq : MATLAB Function  TreatAsAtomicUnit=on
  i_S3abc : Scope  NumInputPorts=3
  i_Sab : Scope  NumInputPorts=2
  psi_Rab : Scope  NumInputPorts=2
  tau_Rcomp : Scope  NumInputPorts=2
  u_S3abc : Scope  NumInputPorts=3
  u_Sab : Scope
  w_R : Scope
  tau_R : Outport
  tag scope: Contr_MI_motor_params=scoped, MI_motor_params=scoped, PBC_params=scoped
  wires:
  [tau_R] -> Bus Creator/1  "tau_R"
  [tau_R] -> tau_R/1
  dq/1 -> [w_R]
  Bus Creator/1 -> To Workspace/1
  [w_R] -> Bus Creator/2  "w_R"
  [u_Sab] -> Bus Creator/3  "u_Sab"
  [i_Sab] -> Bus Creator/4  "i_Sab"
  [u_S3abc] -> Bus Creator/5  "u_S3abc"
  [i_S3abc] -> Bus Creator/6  "i_S3abc"
  [P_elect] -> Bus Creator/7  "P_elect"
  [P_mech] -> Bus Creator/8  "P_mech"
  tau_Rref/1 -> [tau_Rref]
  Product1/1 -> [P_mech]
  Calculo de Potencia eléctrica/3(P_elect) -> [P_elect]
  Demux2/1 -> i_S3abc/1
  [i_Sab] -> Calculo de Potencia eléctrica/2(i_Sab)
  [u_Sab] -> Calculo de Potencia eléctrica/1(u_Sab)
  Calculo de Potencia eléctrica/1(u_S3abc) -> [u_S3abc]
  [tau_R] -> Product1/2
  Demux2/2 -> i_S3abc/2
  Calculo de Potencia eléctrica/2(i_S3abc) -> [i_S3abc]
  [P_mech] -> Potencia/2, Sum2/2
  Sum2/1 -> Potencia/3
  Demux1/2 -> u_S3abc/2
  Demux1/3 -> u_S3abc/3
  Demux1/1 -> u_S3abc/1
  [tau_Rref] -> tau_Rcomp/1
  [w_R] -> Product1/1
  [tau_R] -> tau_Rcomp/2
  [P_elect] -> Potencia/1, Sum2/1
  Demux2/3 -> i_S3abc/3
  [i_S3abc] -> Demux2/1
  [w_R] -> w_R/1
  [u_S3abc] -> Demux1/1
  Modelo MI (modelo ab)/2(dpsi_Rab) -> [psi_Rab]
  Modelo MI (modelo ab)/1(i_Sab) -> Controlador PBC/1(i_Sab), [i_Sab]
  Controlador PBC/1(u_Sref) -> Modelo MI (modelo ab)/1(u_Sab), [u_Sab]
  [tau_Rref] -> Modelo MI (modelo ab)/2(tau_L)
  [w_R] -> Controlador PBC/2(w_R)
  Constant3/1 -> [MI_motor_params]
  [i_Sab] -> Demux5/1
  [psi_Rab] -> Demux6/1
  Demux6/2 -> psi_Rab/2
  Demux5/1 -> i_Sab/1
  Demux5/2 -> i_Sab/2
  [u_Sab] -> u_Sab/1
  [psi_Rab] -> ab/dq/1(f)
  ab/dq/1(f_d) -> Scope6/1
  Demux6/1 -> psi_Rab/1
  Modelo MI (modelo ab)/3(tau_R) -> [tau_R]
  [w_R] -> Modelo MI (modelo ab)/3(w_R)
  Constant5/1 -> [Contr_MI_motor_params]
  Constant4/1 -> [PBC_params]
  ab/dq/2(rho) -> Scope6/2
  [tau_Rref] -> Controlador PBC/3(tau_Rref)

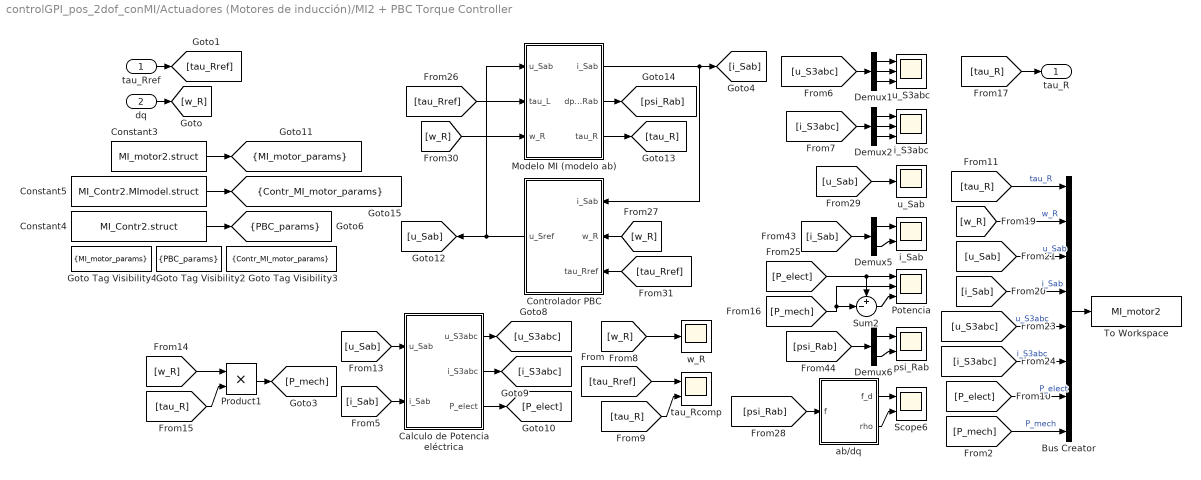
== system controlGPI_pos_2dof_conMI/Actuadores (Motores de inducción)/MI2 + PBC Torque Controller ==
  tau_Rref : Inport
  dq : Inport  Port=2
  Bus Creator : BusCreator  Inputs=8
  Calculo de Potencia eléctrica : Subsystem
  Constant3 : Constant  Value=MI_motor2.struct  OutDataTypeStr=Bus: MI_bus
  Constant4 : Constant  Value=MI_Contr2.struct  OutDataTypeStr=Bus: Contr_bus
  Constant5 : Constant  Value=MI_Contr2.MImodel.struct  OutDataTypeStr=Bus: MI_bus
  Controlador PBC : Subsystem
  Demux1 : Demux  Outputs=3
  Demux2 : Demux  Outputs=3
  Demux5 : Demux  Outputs=2
  Demux6 : Demux  Outputs=2
  Goto Tag Visibility2 : GotoTagVisibility  GotoTag=PBC_params
  Goto Tag Visibility3 : GotoTagVisibility  GotoTag=Contr_MI_motor_params
  Goto Tag Visibility4 : GotoTagVisibility  GotoTag=MI_motor_params
  Modelo MI (modelo ab) : Subsystem
  Potencia : Scope  NumInputPorts=3
  Product1 : Product
  Scope6 : Scope  NumInputPorts=2
  Sum2 : Sum  Inputs=+-|
  To Workspace : ToWorkspace  VariableName=MI_motor2  SaveFormat=Timeseries  SampleTime=-1
  ab/dq : MATLAB Function  TreatAsAtomicUnit=on
  i_S3abc : Scope  NumInputPorts=3
  i_Sab : Scope  NumInputPorts=2
  psi_Rab : Scope  NumInputPorts=2
  tau_Rcomp : Scope  NumInputPorts=2
  u_S3abc : Scope  NumInputPorts=3
  u_Sab : Scope
  w_R : Scope
  tau_R : Outport
  tag scope: Contr_MI_motor_params=scoped, MI_motor_params=scoped, PBC_params=scoped
  wires:
  [tau_R] -> Bus Creator/1  "tau_R"
  [tau_R] -> tau_R/1
  dq/1 -> [w_R]
  Bus Creator/1 -> To Workspace/1
  [w_R] -> Bus Creator/2  "w_R"
  [u_Sab] -> Bus Creator/3  "u_Sab"
  [i_Sab] -> Bus Creator/4  "i_Sab"
  [u_S3abc] -> Bus Creator/5  "u_S3abc"
  [i_S3abc] -> Bus Creator/6  "i_S3abc"
  [P_elect] -> Bus Creator/7  "P_elect"
  [P_mech] -> Bus Creator/8  "P_mech"
  tau_Rref/1 -> [tau_Rref]
  Product1/1 -> [P_mech]
  Calculo de Potencia eléctrica/3(P_elect) -> [P_elect]
  Demux2/1 -> i_S3abc/1
  [i_Sab] -> Calculo de Potencia eléctrica/2(i_Sab)
  [u_Sab] -> Calculo de Potencia eléctrica/1(u_Sab)
  Calculo de Potencia eléctrica/1(u_S3abc) -> [u_S3abc]
  [tau_R] -> Product1/2
  Demux2/2 -> i_S3abc/2
  Calculo de Potencia eléctrica/2(i_S3abc) -> [i_S3abc]
  [P_mech] -> Potencia/2, Sum2/2
  Sum2/1 -> Potencia/3
  Demux1/2 -> u_S3abc/2
  Demux1/3 -> u_S3abc/3
  Demux1/1 -> u_S3abc/1
  [tau_Rref] -> tau_Rcomp/1
  [w_R] -> Product1/1
  [tau_R] -> tau_Rcomp/2
  [P_elect] -> Potencia/1, Sum2/1
  Demux2/3 -> i_S3abc/3
  [i_S3abc] -> Demux2/1
  [w_R] -> w_R/1
  [u_S3abc] -> Demux1/1
  Modelo MI (modelo ab)/2(dpsi_Rab) -> [psi_Rab]
  Modelo MI (modelo ab)/1(i_Sab) -> Controlador PBC/1(i_Sab), [i_Sab]
  Controlador PBC/1(u_Sref) -> Modelo MI (modelo ab)/1(u_Sab), [u_Sab]
  [tau_Rref] -> Modelo MI (modelo ab)/2(tau_L)
  [w_R] -> Controlador PBC/2(w_R)
  Constant3/1 -> [MI_motor_params]
  [i_Sab] -> Demux5/1
  [psi_Rab] -> Demux6/1
  Demux6/2 -> psi_Rab/2
  Demux5/1 -> i_Sab/1
  Demux5/2 -> i_Sab/2
  [u_Sab] -> u_Sab/1
  [psi_Rab] -> ab/dq/1(f)
  ab/dq/1(f_d) -> Scope6/1
  Demux6/1 -> psi_Rab/1
  Modelo MI (modelo ab)/3(tau_R) -> [tau_R]
  [w_R] -> Modelo MI (modelo ab)/3(w_R)
  Constant5/1 -> [Contr_MI_motor_params]
  Constant4/1 -> [PBC_params]
  ab/dq/2(rho) -> Scope6/2
  [tau_Rref] -> Controlador PBC/3(tau_Rref)

== system controlGPI_pos_2dof_conMI/ControladorGPI + NN/2 to 2 (2)1 ==
  In1 : Inport
  In2 : Inport  Port=2
  Demux3 : Demux  Outputs=2
  Demux4 : Demux  Outputs=2
  Mux8 : Mux  Inputs=2
  Mux9 : Mux  Inputs=2
  1 : Outport
  2 : Outport  Port=2
  wires:
  Demux3/1 -> Mux8/1
  Demux3/2 -> Mux9/1
  Mux9/1 -> 2/1
  Demux4/2 -> Mux9/2
  Demux4/1 -> Mux8/2
  Mux8/1 -> 1/1
  In1/1 -> Demux3/1
  In2/1 -> Demux4/1

== system controlGPI_pos_2dof_conMI/ControladorGPI + NN/3 to 6 (3) ==
  In1 : Inport
  In2 : Inport  Port=2
  In3 : Inport  Port=3
  Demux2 : Demux  Outputs=2
  Demux3 : Demux  Outputs=2
  Demux4 : Demux  Outputs=2
  Out1 : Outport
  Out2 : Outport  Port=2
  Out3 : Outport  Port=3
  Out4 : Outport  Port=4
  Out5 : Outport  Port=5
  Out6 : Outport  Port=6
  wires:
  In3/1 -> Demux4/1
  Demux4/1 -> Out3/1
  Demux2/1 -> Out1/1
  Demux3/2 -> Out5/1
  Demux3/1 -> Out2/1
  In1/1 -> Demux2/1
  Demux4/2 -> Out6/1
  Demux2/2 -> Out4/1
  In2/1 -> Demux3/1

== system controlGPI_pos_2dof_conMI/ControladorGPI + NN/Red neuronal ==
  q : Inport
  de_q : Inport  Port=2
  e_p : Inport  Port=3
  B-Spline NNs : Subsystem  TreatAsAtomicUnit=on
  Constant3 : Constant  Value=nn_select
  Constants : Subsystem  TreatAsAtomicUnit=on
  GPI_params : Scope  NumInputPorts=3
  Merge : Merge  Inputs=3
  Merge1 : Merge  Inputs=3
  Merge2 : Merge  Inputs=3
  RBF NNs : Subsystem  TreatAsAtomicUnit=on
  nn_select : Display
  param sintonization selector : If  IfExpression=u1 == 1  ElseIfExpressions=u1 == 2
  Wc : Outport
  Zc : Outport  Port=2
  Pc : Outport  Port=3
  wires:
  param sintonization selector/1 -> B-Spline NNs/Action
  B-Spline NNs/1(Wc) -> Merge/1
  param sintonization selector/3 -> Constants/Action
  Constant3/1 -> nn_select/1, param sintonization selector/1
  B-Spline NNs/2(Zc) -> Merge1/1
  B-Spline NNs/3(Pc) -> Merge2/1
  Constants/1(Wc) -> Merge/2
  Constants/2(Zc) -> Merge1/2
  Constants/3(Pc) -> Merge2/2
  q/1 -> [e_q]
  de_q/1 -> [de_q]
  param sintonization selector/2 -> RBF NNs/Action
  RBF NNs/2(Zc) -> Merge1/3
  RBF NNs/1(Wc) -> Merge/3
  RBF NNs/3(Pc) -> Merge2/3
  Merge/1 -> GPI_params/1, Wc/1
  Merge1/1 -> GPI_params/2, Zc/1
  Merge2/1 -> GPI_params/3, Pc/1
  [e_q] -> B-Spline NNs/1(e_q)
  [de_q] -> B-Spline NNs/2(de_q)
  [e_q] -> RBF NNs/1(e_q)
  [de_q] -> RBF NNs/2(de_q)
  e_p/1 -> [e_p]
  [e_p] -> RBF NNs/3(e_p)
  [e_p] -> B-Spline NNs/3(e_p)

== system controlGPI_pos_2dof_conMI/Perfil torque de carga tau_L/If Action Subsystem ==
  perfil_params : Inport
  Action Port : ActionPort
  Clock2 : Clock
  Clock4 : Clock
  Polinomio 7mo orden sen : MATLAB Function  TreatAsAtomicUnit=on
  Scope1 : Scope
  Scope4 : Scope
  Scope5 : Scope  NumInputPorts=4
  Senoidal tiempo de inicio : MATLAB Function  TreatAsAtomicUnit=on
  Sum1 : Sum  Inputs=|-+
  senoidal : Sin  TimeSource=Use external signal  Frequency=6.2832  Phase=1.5708  SampleTime=0
  sen : Outport
  wires:
  Clock4/1 -> Polinomio 7mo orden sen/1(t)
  Polinomio 7mo orden sen/1(qpol) -> Scope1/1, Sum1/1, Scope5/1
  Sum1/1 -> Scope4/1, [sen]
  Polinomio 7mo orden sen/4(jpol) -> Scope5/4
  Polinomio 7mo orden sen/3(apol) -> Scope5/3
  Clock2/1 -> Senoidal tiempo de inicio/1(t)
  [perfil_params] -> Polinomio 7mo orden sen/2(perfil_params)
  Polinomio 7mo orden sen/2(vpol) -> Scope5/2
  senoidal/1 -> Sum1/2
  Senoidal tiempo de inicio/1(tr) -> senoidal/1
  [sen] -> sen/1
  perfil_params/1 -> [perfil_params]
  [perfil_params] -> Senoidal tiempo de inicio/2(perfil_params)

== system controlGPI_pos_2dof_conMI/Perfil torque de carga tau_L/If Action Subsystem1 ==
  Action Port : ActionPort
  Constant : Constant  Value=0
  cero : Outport
  wires:
  Constant/1 -> cero/1

== system controlGPI_pos_2dof_conMI/Perfil torque de carga tau_L/If Action Subsystem2 ==
  Action Port : ActionPort
  Scope3 : Scope
  Sum : Sum  Inputs=|++
  escalon1 : Step  Time=2.5  After=0.70582  SampleTime=0
  escalon2 : Step  Time=7.5  After=-0.70582  SampleTime=0
  esca : Outport
  wires:
  escalon2/1 -> Sum/2
  escalon1/1 -> Sum/1
  Sum/1 -> [esca], Scope3/1
  [esca] -> esca/1

== system controlGPI_pos_2dof_conMI/Perfil torque de carga tau_L/If Action Subsystem3 ==
  Action Port : ActionPort
  Scope2 : Scope
  Sum2 : Sum  Inputs=|++
  rampa1 : simulink/Sources/Ramp  slope=0.02064  start=2.5  InitialOutput=0
  rampa2 : simulink/Sources/Ramp  slope=-0.02064  start=7.5  InitialOutput=0
  ramp : Outport
  wires:
  rampa2/1 -> Sum2/2
  rampa1/1 -> Sum2/1
  Sum2/1 -> Scope2/1, [ramp]
  [ramp] -> ramp/1

== system controlGPI_pos_2dof_conMI/Perfil torque de carga tau_L/If Action Subsystem4 ==
  perfil_params : Inport
  Action Port : ActionPort
  Clock1 : Clock
  Polinomio 7mo orden tau_L : MATLAB Function  TreatAsAtomicUnit=on
  Scope : Scope  NumInputPorts=4
  pol7 : Outport
  wires:
  Polinomio 7mo orden tau_L/4(jpol) -> Scope/4
  Polinomio 7mo orden tau_L/1(qpol) -> Scope/1, [pol7]
  Polinomio 7mo orden tau_L/2(vpol) -> Scope/2
  Clock1/1 -> Polinomio 7mo orden tau_L/1(t)
  Polinomio 7mo orden tau_L/3(apol) -> Scope/3
  perfil_params/1 -> Polinomio 7mo orden tau_L/2(perfil_params)
  [pol7] -> pol7/1

== system controlGPI_pos_2dof_conMI/Perfil torque de carga tau_L/If Action Subsystem5 ==
  perfil_params : Inport
  Action Port : ActionPort
  Clock : Clock
  Scope1 : Scope
  Tren de esca : MATLAB Function  TreatAsAtomicUnit=on
  trEsca : Outport
  wires:
  Tren de esca/1(q) -> Scope1/1, [trEsca]
  Clock/1 -> Tren de esca/1(t)
  perfil_params/1 -> Tren de esca/2(perfil_params)
  [trEsca] -> trEsca/1

== system controlGPI_pos_2dof_conMI/Perfil torque de carga tau_L/If Action Subsystem6 ==
  Action Port : ActionPort
  Clock3 : Clock
  Polinomio 7mo orden timeseries : MATLAB Function  TreatAsAtomicUnit=on
  Product : Product
  Scope6 : Scope  NumInputPorts=4
  ts_data1 : FromWorkspace  Commented=on  VariableName=tau_L_ts
  ts : Outport
  wires:
  Product/1 -> [ts]
  Clock3/1 -> Polinomio 7mo orden timeseries/1(t)
  ts_data1/1 -> Product/1
  Polinomio 7mo orden timeseries/4(jpol) -> Scope6/4
  Polinomio 7mo orden timeseries/2(vpol) -> Scope6/2
  Polinomio 7mo orden timeseries/3(apol) -> Scope6/3
  Polinomio 7mo orden timeseries/1(qpol) -> Product/2, Scope6/1
  [ts] -> ts/1

== system controlGPI_pos_2dof_conMI/Perfil torque de carga tau_L/If Action Subsystem7 ==
  perfil_params : Inport
  Action Port : ActionPort
  Clock5 : Clock
  Scope7 : Scope
  Trayectoria 15 segmentos : MATLAB Function  TreatAsAtomicUnit=on
  tr15segs : Outport
  wires:
  Clock5/1 -> Trayectoria 15 segmentos/1(t)
  Trayectoria 15 segmentos/1(q) -> Scope7/1, [tr15segs]
  [tr15segs] -> tr15segs/1
  perfil_params/1 -> Trayectoria 15 segmentos/2(perfil_params)

== system controlGPI_pos_2dof_conMI/Trayectoria de referencia/2 to 2 (2) ==
  In1 : Inport
  In2 : Inport  Port=2
  Demux3 : Demux  Outputs=2
  Demux4 : Demux  Outputs=2
  Mux8 : Mux  Inputs=2
  Mux9 : Mux  Inputs=2
  1 : Outport
  2 : Outport  Port=2
  wires:
  Demux3/1 -> Mux8/1
  Demux3/2 -> Mux9/1
  Mux9/1 -> 2/1
  Demux4/2 -> Mux9/2
  Demux4/1 -> Mux8/2
  Mux8/1 -> 1/1
  In1/1 -> Demux3/1
  In2/1 -> Demux4/1

== system controlGPI_pos_2dof_conMI/Trayectoria de referencia/2 to 2 (2)1 ==
  In1 : Inport
  In2 : Inport  Port=2
  Demux3 : Demux  Outputs=2
  Demux4 : Demux  Outputs=2
  Mux8 : Mux  Inputs=2
  Mux9 : Mux  Inputs=2
  1 : Outport
  2 : Outport  Port=2
  wires:
  Demux3/1 -> Mux8/1
  Demux3/2 -> Mux9/1
  Mux9/1 -> 2/1
  Demux4/2 -> Mux9/2
  Demux4/1 -> Mux8/2
  Mux8/1 -> 1/1
  In1/1 -> Demux3/1
  In2/1 -> Demux4/1

== system controlGPI_pos_2dof_conMI/Trayectoria de referencia/2 to 2 (2)2 ==
  In1 : Inport
  In2 : Inport  Port=2
  Demux3 : Demux  Outputs=2
  Demux4 : Demux  Outputs=2
  Mux8 : Mux  Inputs=2
  Mux9 : Mux  Inputs=2
  1 : Outport
  2 : Outport  Port=2
  wires:
  Demux3/1 -> Mux8/1
  Demux3/2 -> Mux9/1
  Mux9/1 -> 2/1
  Demux4/2 -> Mux9/2
  Demux4/1 -> Mux8/2
  Mux8/1 -> 1/1
  In1/1 -> Demux3/1
  In2/1 -> Demux4/1

== system controlGPI_pos_2dof_conMI/Trayectoria de referencia/3 to 6 (4) ==
  In1 : Inport
  In2 : Inport  Port=2
  In3 : Inport  Port=3
  Demux2 : Demux  Outputs=2
  Demux3 : Demux  Outputs=2
  Demux4 : Demux  Outputs=2
  Out1 : Outport
  Out2 : Outport  Port=2
  Out3 : Outport  Port=3
  Out4 : Outport  Port=4
  Out5 : Outport  Port=5
  Out6 : Outport  Port=6
  wires:
  In3/1 -> Demux4/1
  Demux4/1 -> Out3/1
  Demux2/1 -> Out1/1
  Demux3/2 -> Out5/1
  Demux3/1 -> Out2/1
  In1/1 -> Demux2/1
  Demux4/2 -> Out6/1
  Demux2/2 -> Out4/1
  In2/1 -> Demux3/1

== system controlGPI_pos_2dof_conMI/Trayectoria de referencia/3 to 6 (4)1 ==
  In1 : Inport
  In2 : Inport  Port=2
  In3 : Inport  Port=3
  Demux2 : Demux  Outputs=2
  Demux3 : Demux  Outputs=2
  Demux4 : Demux  Outputs=2
  Out1 : Outport
  Out2 : Outport  Port=2
  Out3 : Outport  Port=3
  Out4 : Outport  Port=4
  Out5 : Outport  Port=5
  Out6 : Outport  Port=6
  wires:
  In3/1 -> Demux4/1
  Demux4/1 -> Out3/1
  Demux2/1 -> Out1/1
  Demux3/2 -> Out5/1
  Demux3/1 -> Out2/1
  In1/1 -> Demux2/1
  Demux4/2 -> Out6/1
  Demux2/2 -> Out4/1
  In2/1 -> Demux3/1

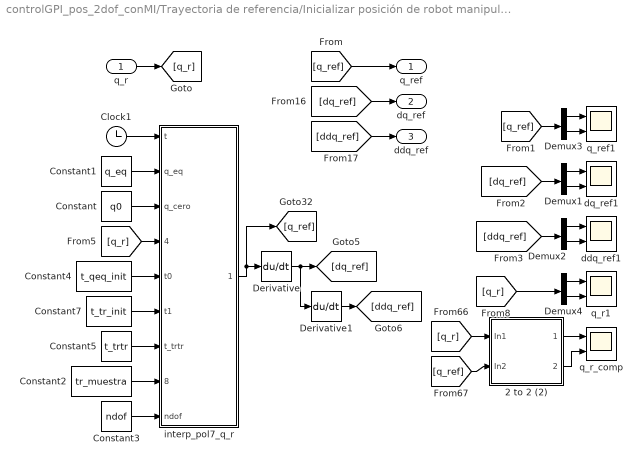
== system controlGPI_pos_2dof_conMI/Trayectoria de referencia/Inicializar posición de robot manipulador ==
  q_r : Inport
  2 to 2 (2) : Subsystem
  Clock1 : Clock
  Constant : Constant  Value=q0
  Constant1 : Constant  Value=q_eq
  Constant2 : Constant  Value=tr_muestra
  Constant3 : Constant  Value=ndof
  Constant4 : Constant  Value=t_qeq_init
  Constant5 : Constant  Value=t_trtr
  Constant7 : Constant  Value=t_tr_init
  Demux{1..4} (4 alike) : Demux  Outputs=2
  Derivative : Derivative
  Derivative1 : Derivative
  ddq_ref1 : Scope  NumInputPorts=2
  dq_ref1 : Scope  NumInputPorts=2
  interp_pol7_q_r : MATLAB Function  TreatAsAtomicUnit=on
  q_r1 : Scope  NumInputPorts=2
  q_r_comp : Scope  NumInputPorts=2
  q_ref1 : Scope  NumInputPorts=2
  q_ref : Outport
  dq_ref : Outport  Port=2
  ddq_ref : Outport  Port=3
  wires:
  [ddq_ref] -> ddq_ref/1
  q_r/1 -> [q_r]
  [dq_ref] -> dq_ref/1
  [q_ref] -> q_ref/1
  [q_r] -> 2 to 2 (2)/1(In1)
  [q_ref] -> 2 to 2 (2)/2(In2)
  [q_r] -> Demux4/1
  interp_pol7_q_r/1(interp_qpos) -> [q_ref], Derivative/1
  Derivative/1 -> [dq_ref], Derivative1/1
  Derivative1/1 -> [ddq_ref]
  [q_ref] -> Demux3/1
  [dq_ref] -> Demux1/1
  [ddq_ref] -> Demux2/1
  Constant5/1 -> interp_pol7_q_r/7(t_trtr)
  Constant4/1 -> interp_pol7_q_r/5(t0)
  Constant1/1 -> interp_pol7_q_r/2(q_eq)
  [q_r] -> interp_pol7_q_r/4(q_tr_init)
  Constant3/1 -> interp_pol7_q_r/9(ndof)
  Constant/1 -> interp_pol7_q_r/3(q_cero)
  Clock1/1 -> interp_pol7_q_r/1(t)
  Constant7/1 -> interp_pol7_q_r/6(t1)
  Constant2/1 -> interp_pol7_q_r/8(tr_muestra)
  Demux3/1 -> q_ref1/1
  Demux3/2 -> q_ref1/2
  Demux1/1 -> dq_ref1/1
  Demux1/2 -> dq_ref1/2
  Demux2/1 -> ddq_ref1/1
  Demux2/2 -> ddq_ref1/2
  Demux4/1 -> q_r1/1
  Demux4/2 -> q_r1/2
  2 to 2 (2)/1(1) -> q_r_comp/1
  2 to 2 (2)/2(2) -> q_r_comp/2

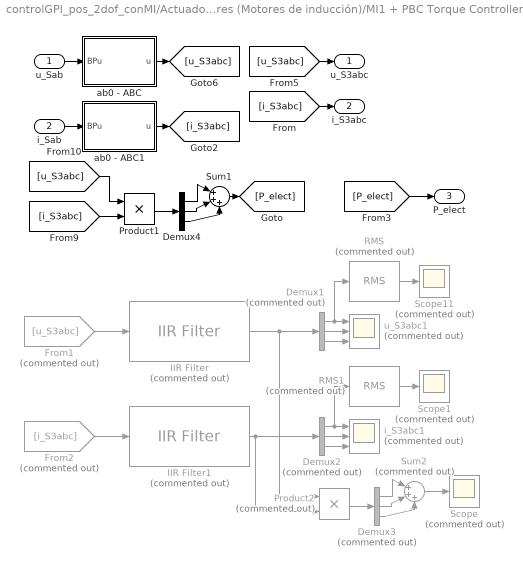
== system controlGPI_pos_2dof_conMI/Actuadores (Motores de inducción)/MI1 + PBC Torque Controller/Calculo de Potencia eléctrica ==
  u_Sab : Inport
  i_Sab : Inport  Port=2
  Demux1 : Demux  Commented=on  Outputs=3
  Demux2 : Demux  Commented=on  Outputs=3
  Demux3 : Demux  Commented=on  Outputs=3
  Demux4 : Demux  Outputs=3
  From1 : From  Commented=on  GotoTag=u_S3abc
  From2 : From  Commented=on  GotoTag=i_S3abc
  IIR Filter : mcbcontrolslib/IIR Filter  Commented=on  VariantControl=Low Pass Filter  VariantSelect=Low-pass  Filter_constant=0.04  advancedSettings=on  Ts=50e-6  cutOff_freq=132.6291
      settings: LibrarySourceBlock=mcbhdllib/Signal Management/IIR Filter
  IIR Filter1 : mcbcontrolslib/IIR Filter  Commented=on  VariantControl=Low Pass Filter  VariantSelect=Low-pass  Filter_constant=0.04  advancedSettings=on  Ts=50e-6  cutOff_freq=132.6291
      settings: LibrarySourceBlock=mcbhdllib/Signal Management/IIR Filter
  Product1 : Product
  Product2 : Product  Commented=on
  RMS : spsRMSLib/RMS  Commented=on  TrueRMS=on  Freq=60  RMSInit=120  Ts=0
  RMS1 : spsRMSLib/RMS  Commented=on  TrueRMS=on  Freq=60  RMSInit=120  Ts=0
  Scope : Scope  Commented=on
  Scope1 : Scope  Commented=on
  Scope11 : Scope  Commented=on
  Sum1 : Sum  Inputs=|+++
  Sum2 : Sum  Commented=on  Inputs=|+++
  ab0 - ABC : MATLAB Function  TreatAsAtomicUnit=on
  ab0 - ABC1 : MATLAB Function  TreatAsAtomicUnit=on
  i_S3abc1 : Scope  Commented=on  NumInputPorts=3
  u_S3abc1 : Scope  Commented=on  NumInputPorts=3
  u_S3abc : Outport
  i_S3abc : Outport  Port=2
  P_elect : Outport  Port=3
  wires:
  Demux4/1 -> Sum1/1
  [i_S3abc] -> Product1/2
  i_Sab/1 -> ab0 - ABC1/1(BPu)
  Demux4/3 -> Sum1/3
  [u_S3abc] -> Product1/1
  Demux4/2 -> Sum1/2
  Product1/1 -> Demux4/1
  u_Sab/1 -> ab0 - ABC/1(BPu)
  [u_S3abc] -> u_S3abc/1
  [i_S3abc] -> i_S3abc/1
  ab0 - ABC/1(u) -> [u_S3abc]
  ab0 - ABC1/1(u) -> [i_S3abc]
  IIR Filter/1 -> Product2/1, Demux1/1
  RMS/1 -> Scope11/1
  Demux1/2 -> u_S3abc1/2
  Demux1/3 -> u_S3abc1/3
  Demux1/1 -> RMS/1, u_S3abc1/1
  From1/1 -> IIR Filter/1
  Demux2/1 -> RMS1/1, i_S3abc1/1
  RMS1/1 -> Scope1/1
  Demux2/2 -> i_S3abc1/2
  IIR Filter1/1 -> Product2/2, Demux2/1
  From2/1 -> IIR Filter1/1
  Demux2/3 -> i_S3abc1/3
  Demux3/2 -> Sum2/2
  Demux3/3 -> Sum2/3
  Sum2/1 -> Scope/1
  Product2/1 -> Demux3/1
  Demux3/1 -> Sum2/1
  Sum1/1 -> [P_elect]
  [P_elect] -> P_elect/1

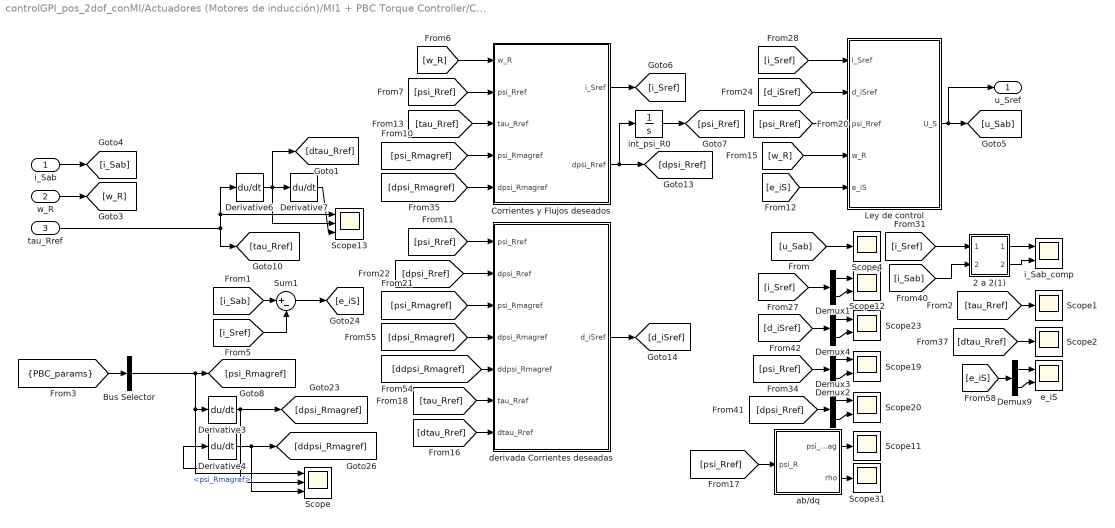
== system controlGPI_pos_2dof_conMI/Actuadores (Motores de inducción)/MI1 + PBC Torque Controller/Controlador PBC ==
  i_Sab : Inport
  w_R : Inport  Port=2
  tau_Rref : Inport  Port=3
  2 a 2(1) : Subsystem
  Bus Selector : BusSelector  OutputSignals=psi_Rmagref
  Corrientes y Flujos deseados : Subsystem
  Demux{1..4,9} (5 alike) : Demux  Outputs=2
  Derivative{3..4,6..7} (4 alike) : Derivative
  Ley de control : Subsystem
  Scope : Scope  NumInputPorts=3
  Scope{1..2,4,11,31} (5 alike) : Scope
  Scope{12,19..20,23} (4 alike) : Scope  NumInputPorts=2
  Scope13 : Scope  NumInputPorts=3
  Sum1 : Sum  Inputs=|+-
  ab/dq : MATLAB Function  TreatAsAtomicUnit=on
  derivada Corrientes deseadas : Subsystem
  e_iS : Scope  NumInputPorts=2
  i_Sab_comp : Scope  NumInputPorts=2
  int_psi_R0 : Integrator  InitialCondition=[0.51032;0]
  u_Sref : Outport
  wires:
  Derivative3/1 -> Scope/2, Derivative4/1, [dpsi_Rmagref]
  Derivative4/1 -> [ddpsi_Rmagref], Scope/3
  Bus Selector/1 -> Scope/1, Derivative3/1, [psi_Rmagref]  "<psi_Rmagref>"
  i_Sab/1 -> [i_Sab]
  [tau_Rref] -> Corrientes y Flujos deseados/3(tau_Rref)
  [w_R] -> Corrientes y Flujos deseados/1(w_R)
  int_psi_R0/1 -> [psi_Rref]
  Corrientes y Flujos deseados/2(dpsi_Rref) -> int_psi_R0/1, [dpsi_Rref]
  [psi_Rref] -> Corrientes y Flujos deseados/2(psi_Rref)
  [psi_Rmagref] -> Corrientes y Flujos deseados/4(psi_Rmagref)
  [dpsi_Rmagref] -> Corrientes y Flujos deseados/5(dpsi_Rmagref)
  [psi_Rref] -> derivada Corrientes deseadas/1(psi_Rref)
  [dpsi_Rref] -> derivada Corrientes deseadas/2(dpsi_Rref)
  [psi_Rmagref] -> derivada Corrientes deseadas/3(psi_Rmagref)
  [dpsi_Rmagref] -> derivada Corrientes deseadas/4(dpsi_Rmagref)
  [ddpsi_Rmagref] -> derivada Corrientes deseadas/5(ddpsi_Rmagref)
  [tau_Rref] -> derivada Corrientes deseadas/6(tau_Rref)
  [dtau_Rref] -> derivada Corrientes deseadas/7(dtau_Rref)
  derivada Corrientes deseadas/1(d_iSref) -> [d_iSref]
  [e_iS] -> Demux9/1
  Demux9/1 -> e_iS/1
  Demux9/2 -> e_iS/2
  [i_Sab] -> Sum1/1
  [i_Sref] -> Sum1/2
  Sum1/1 -> [e_iS]
  [i_Sref] -> Ley de control/1(i_Sref)
  [d_iSref] -> Ley de control/2(d_iSref)
  [psi_Rref] -> Ley de control/3(psi_Rref)
  [w_R] -> Ley de control/4(w_R)
  Ley de control/1(U_S) -> u_Sref/1, [u_Sab]
  [e_iS] -> Ley de control/5(e_iS)
  Derivative7/1 -> Scope13/3
  Derivative6/1 -> [dtau_Rref], Derivative7/1, Scope13/2
  2 a 2(1)/2(Out2) -> i_Sab_comp/2
  2 a 2(1)/1(Out1) -> i_Sab_comp/1
  [i_Sab] -> 2 a 2(1)/2(In2)
  [i_Sref] -> 2 a 2(1)/1(In1)
  w_R/1 -> [w_R]
  [tau_Rref] -> Scope1/1
  [PBC_params] -> Bus Selector/1
  Corrientes y Flujos deseados/1(i_Sref) -> [i_Sref]
  tau_Rref/1 -> [tau_Rref], Derivative6/1, Scope13/1
  ab/dq/1(psi_Rmag) -> Scope11/1
  ab/dq/2(rho) -> Scope31/1
  [psi_Rref] -> ab/dq/1(psi_R)
  Demux4/1 -> Scope23/1
  [i_Sref] -> Demux1/1
  [u_Sab] -> Scope4/1
  Demux2/2 -> Scope19/2
  [psi_Rref] -> Demux2/1
  Demux3/2 -> Scope20/2
  Demux3/1 -> Scope20/1
  [d_iSref] -> Demux4/1
  Demux4/2 -> Scope23/2
  Demux2/1 -> Scope19/1
  [dpsi_Rref] -> Demux3/1
  Demux1/2 -> Scope12/2
  Demux1/1 -> Scope12/1
  [dtau_Rref] -> Scope2/1
